simulink model "BaseFahrzeug_KonEffEM"  (R2013a)
settings: Solver=ode5  StartTime=0.0  StopTime=max(sim_sample_time)  FixedStep=0.01  RelTol=1e-3
values from neighbouring files (symbols this model uses):
  drive_acc =     [NoGenDoubleNEDC.mat]
  PwpPt_Tq_EngGross = [0 0 0 1.18647349782e-14 1.38134887733e-14 1.57622425684e-14 1.77109963635e-14 1.96597501586e-14 2.16085039538e-14 2.35572577489e-14 2.5506011544e-14 2.74547653391e-14 ... (23602 elements, 23602x1)]    [NoGenDoubleNEDC.mat]    (also in newdoublecycle.m = [PwpPt_Tq_EngGross;PwpPt_Tq_EngGross])
  PwpPt_W_EngDn = [750 750 750 750 750 750 750 750 750 750 750 750 ... (23602 elements, 23602x1)]    [NoGenDoubleNEDC.mat]    (also in newdoublecycle.m = [PwpPt_W_EngDn;PwpPt_W_EngDn])
  sim_sample_time = [0 0.1 0.2 0.3 0.4 0.5 0.6 0.7 0.8 0.9 1 1.1 ... (23602 elements, 23602x1)]    [NoGenDoubleNEDC.mat]    (also in newdoublecycle.m = [sim_sample_time;sim_sample_time+max(sim_sample_time)+0.1])
undefined symbols (not defined in the file or in its folder): KonstEMWirk, PEEM
undefined symbols (not defined in the file): engine
settings Model: Creator=meifert  LastModifiedBy=meifert
settings DataIOCC: SignalLoggingSaveFormat=ModelDataLogs
settings OptimizationCC: BooleanDataType=off
settings DebuggingCC: SaveWithParameterizedLinksMsg=none  SignalResolutionControl=TryResolveAllWithWarning  SolverPrmCheckMsg=none  MultiTaskDSMMsg=warning  MultiTaskCondExecSysMsg=none  StrictBusMsg=None
settings HardwareCC: TargetUnknown=on
settings RTWCC: IncludeERTFirstTime=on
settings GRTTargetCC: CombineOutputUpdateFcns=off  GRTInterface=on

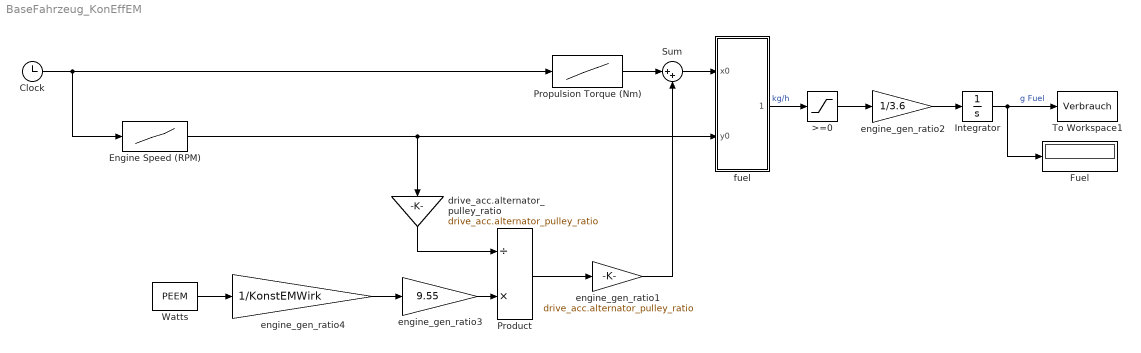
== system BaseFahrzeug_KonEffEM ==
  >=0 : Saturate  UpperLimit=inf  LowerLimit=0
  Clock : Clock
  Engine Speed (RPM) : Lookup  InputValues=sim_sample_time  Table=PwpPt_W_EngDn  SaturateOnIntegerOverflow=on
  Fuel : Display
  Integrator : Integrator
  Product : Product  Inputs=/*
  Propulsion Torque (Nm) : Lookup  InputValues=sim_sample_time  Table=PwpPt_Tq_EngGross  SaturateOnIntegerOverflow=on
  Sum : Sum  Inputs=|++  SaturateOnIntegerOverflow=on  InputSameDT=on  OutDataTypeStr=Inherit: Same as first input
  To Workspace1 : ToWorkspace  VariableName=Verbrauch  SampleTime=-1
  Watts : Constant  Value=PEEM
  drive_acc.alternator_pulley_ratio : Gain  Gain=drive_acc.alternator_pulley_ratio  SaturateOnIntegerOverflow=on  OutDataTypeStr=Inherit: Same as input  ParamDataTypeStr=Inherit: Same as input
  engine_gen_ratio1 : Gain  Gain=drive_acc.alternator_pulley_ratio  SaturateOnIntegerOverflow=on  OutDataTypeStr=Inherit: Same as input  ParamDataTypeStr=Inherit: Same as input
  engine_gen_ratio2 : Gain  Gain=1/3.6  SaturateOnIntegerOverflow=on  OutDataTypeStr=Inherit: Same as input  ParamDataTypeStr=Inherit: Same as input
  engine_gen_ratio3 : Gain  Gain=9.55  SaturateOnIntegerOverflow=on  OutDataTypeStr=Inherit: Same as input  ParamDataTypeStr=Inherit: Same as input
  engine_gen_ratio4 : Gain  Gain=1/KonstEMWirk  SaturateOnIntegerOverflow=on  OutDataTypeStr=Inherit: Same as input  ParamDataTypeStr=Inherit: Same as input
  fuel : Subsystem  mask(2-D Table Lookup){xindex=engine.tq, yindex=engine.rpm, table=engine.fuel}
      mask prompts: xindex "X Index"; yindex "Y Index"
      mask help:
      | Two Dimensional Table Lookup
      | The first input corresponds to X Index and the second input corresponds to the Y Index
      mask init:
      | sftab2chk(xindex,yindex,table);
      mask Help: This block returns a linearly interpolated intersection from the table using the X index (which corresponds to the rows of the table) and the Y index (which corresponds to the columns of the table).  Extrapolation is used.
      mask Display: plot(-10,-10,110,110,[90,50,10],[90,40,30],[90,50,10],[50,26,20],[90,50,10],[22,13,10])
  wires:
  Integrator/1 -> To Workspace1/1, Fuel/1  "g Fuel"
  fuel/1(table out) -> >=0/1  "kg/h"
  >=0/1 -> engine_gen_ratio2/1
  Clock/1 -> Engine Speed (RPM)/1, Propulsion Torque (Nm)/1
  Engine Speed (RPM)/1 -> fuel/2(y0), drive_acc.alternator_pulley_ratio/1
  Product/1 -> engine_gen_ratio1/1
  engine_gen_ratio1/1 -> Sum/2
  Propulsion Torque (Nm)/1 -> Sum/1
  engine_gen_ratio2/1 -> Integrator/1
  Sum/1 -> fuel/1(x0)
  drive_acc.alternator_pulley_ratio/1 -> Product/1
  engine_gen_ratio4/1 -> engine_gen_ratio3/1
  Watts/1 -> engine_gen_ratio4/1
  engine_gen_ratio3/1 -> Product/2

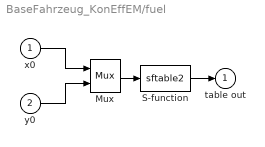
== system BaseFahrzeug_KonEffEM/fuel ==
  x0 : Inport
  y0 : Inport  Port=2
  Mux : Mux  Inputs=2
  S-function : S-Function  FunctionName=sftable2  Parameters=xindex, yindex, table  EnableBusSupport=off
  table out : Outport  InitialOutput=0
  wires:
  Mux/1 -> S-function/1
  x0/1 -> Mux/1
  S-function/1 -> table out/1
  y0/1 -> Mux/2
